simulink model "mrefrobotarm_previous_y_previous_u_previous_ref_cex_2"  (R2018b)
settings: Solver=FixedStepAuto  StartTime=0.0  StopTime=20  RelTol=1e-3  AbsTol=1e-6
undefined symbols (not defined in the file or in its folder): cc, options
libraries: neural x462, simulink x2
(part 16 of 18)

== system mrefrobotarm_previous_y_previous_u_previous_ref_cex_2/no_cex1/Layer 3/Delays 1 ==
  "p{3}" : Inport  PortDimensions=30
      mask Display: e = 0.06;c1 = [120 230 180]/255;c2 = ([120 230 180]+0)/(256+128);c3 = ([120 230 180]+128)/(256+128);patch([0 1 1 0],[0 0 1 1],c1);patch([0 1 1 1-e 1-e 0+e],[0 0 1 1-e 0+e 0+e],c2);patch([0 0 1 1-e 0+e 0+e],[0 1 1 1-e 1-e 0+e],c3);plot([0 1 1 0 0],[0 0 1 1 0]);
  mux : Mux  Inputs=1
      mask Display: e = 0.06;c1 = [120 150 230]/255;c2 = ([120 150 230]+0)/383;c3 = ([120 150 230]+128)/383;patch([0 1 1 0],[0 0 1 1],c1);patch([0 1 1 1-e 1-e 0+e],[0 0 1 1-e 0+e 0+e],c2);patch([0 0 1 1-e 0+e 0+e],[0 1 1 1-e 1-e 0+e],c3);plot([0 1 1 0 0],[0 0 1 1 0]);disp('Mux')
  "pd{3,2}" : Outport
      mask Display: e = 0.06;c1 = [120 230 180]/255;c2 = ([120 230 180]+0)/(256+128);c3 = ([120 230 180]+128)/(256+128);patch([0 1 1 0],[0 0 1 1],c1);patch([0 1 1 1-e 1-e 0+e],[0 0 1 1-e 0+e 0+e],c2);patch([0 0 1 1-e 0+e 0+e],[0 1 1 1-e 1-e 0+e],c3);plot([0 1 1 0 0],[0 0 1 1 0]);
  wires:
  "p{3}"/1 -> mux/1
  mux/1 -> "pd{3,2}"/1

== system mrefrobotarm_previous_y_previous_u_previous_ref_cex_2/no_cex1/Layer 3/LW{3,2} ==
  "ad{3,2}" : Inport  PortDimensions=30
      mask Display: e = 0.06;c1 = [120 230 180]/255;c2 = ([120 230 180]+0)/(256+128);c3 = ([120 230 180]+128)/(256+128);patch([0 1 1 0],[0 0 1 1],c1);patch([0 1 1 1-e 1-e 0+e],[0 0 1 1-e 0+e 0+e],c2);patch([0 0 1 1-e 0+e 0+e],[0 1 1 1-e 1-e 0+e],c3);plot([0 1 1 0 0],[0 0 1 1 0]);
  "IW{3,2}(1,:)'" : Constant  Value=[-0.179633159964680266806880126750911585986614227294921875;-0.01072873765062364037614628387018456123769283294677734375;-0.0291453057248748058360998669513719505630433559417724609375;0.05859045612955075810202032471352140419185161590576171875;-0.237638764700321913903025006220559589564800262451171875;-0.209838527725091539277713081901310943067073822021484375;-0.27791655307496510030063063823035918176174163818359375;-0.07008976059233355815347721318175899796187877655029296875;-0.11554327471293225626514100667918683029711246490478515625;0.27212249906517038677833397741778753697872161865234375;-0.1734031338030869451305449047140427865087985992431640625;0.0536763624525791460673218580268439836800098419189453125;-0.037173437880853761605681739865758572705090045928955078125;0.1358518131119930971717479906146763823926448822021484375;-0.11157815841815578450368917629020870663225650787353515625;-0.023913464068717076027592582931902143172919750213623046875;-0.4313994517536372530486232790281064808368682861328125;0.1636875861604869808463291747102630324661731719970703125;0.037232113811342650022684352961732656694948673248291015625;-0.52644415726454052428806562602403573691844940185546875;0.039897217969779720514456045066253864206373691558837890625;-0.1369287872106144388073545314910006709396839141845703125;0.44593864887069745162051503939437679946422576904296875;0.410742338437982856813590615274733863770961761474609375;-0.145121658875231818175421949490555562078952789306640625;0.06655502995710448066457587401600903831422328948974609375;-0.418109406113754300537976860141498036682605743408203125;0.11096998879556761730125202802810235880315303802490234375;0.333827163986122277261614499366260133683681488037109375;0.186101897373585012385177606120123527944087982177734375]
      mask Display: e = 0.06;c1 = [120 150 230]/255;c2 = ([120 150 230]+0)/383;c3 = ([120 150 230]+128)/383;patch([0 1 1 0],[0 0 1 1],c1);patch([0 1 1 1-e 1-e 0+e],[0 0 1 1-e 0+e 0+e],c2);patch([0 0 1 1-e 0+e 0+e],[0 1 1 1-e 1-e 0+e],c3);plot([0 1 1 0 0],[0 0 1 1 0]);disp('weights');
  Mux : Mux  Inputs=1
      mask Display: e = 0.06;c1 = [120 150 230]/255;c2 = ([120 150 230]+0)/383;c3 = ([120 150 230]+128)/383;patch([0 1 1 0],[0 0 1 1],c1);patch([0 1 1 1-e 1-e 0+e],[0 0 1 1-e 0+e 0+e],c2);patch([0 0 1 1-e 0+e 0+e],[0 1 1 1-e 1-e 0+e],c3);plot([0 1 1 0 0],[0 0 1 1 0]);disp('Mux');
  dotprod1 : neural/Weight Functions/dotprod
  "lz{3,2}" : Outport
      mask Display: e = 0.06;c1 = [120 230 180]/255;c2 = ([120 230 180]+0)/(256+128);c3 = ([120 230 180]+128)/(256+128);patch([0 1 1 0],[0 0 1 1],c1);patch([0 1 1 1-e 1-e 0+e],[0 0 1 1-e 0+e 0+e],c2);patch([0 0 1 1-e 0+e 0+e],[0 1 1 1-e 1-e 0+e],c3);plot([0 1 1 0 0],[0 0 1 1 0]);
  wires:
  "IW{3,2}(1,:)'"/1 -> dotprod1/1
  "ad{3,2}"/1 -> dotprod1/2
  dotprod1/1 -> Mux/1
  Mux/1 -> "lz{3,2}"/1

== system mrefrobotarm_previous_y_previous_u_previous_ref_cex_2/no_cex_old/Layer 1/Delays 1 ==
  "p{1}" : Inport  PortDimensions=10
      mask Display: e = 0.06;c1 = [120 230 180]/255;c2 = ([120 230 180]+0)/(256+128);c3 = ([120 230 180]+128)/(256+128);patch([0 1 1 0],[0 0 1 1],c1);patch([0 1 1 1-e 1-e 0+e],[0 0 1 1-e 0+e 0+e],c2);patch([0 0 1 1-e 0+e 0+e],[0 1 1 1-e 1-e 0+e],c3);plot([0 1 1 0 0],[0 0 1 1 0]);
  mux : Mux  Inputs=1
      mask Display: e = 0.06;c1 = [120 150 230]/255;c2 = ([120 150 230]+0)/383;c3 = ([120 150 230]+128)/383;patch([0 1 1 0],[0 0 1 1],c1);patch([0 1 1 1-e 1-e 0+e],[0 0 1 1-e 0+e 0+e],c2);patch([0 0 1 1-e 0+e 0+e],[0 1 1 1-e 1-e 0+e],c3);plot([0 1 1 0 0],[0 0 1 1 0]);disp('Mux')
  "pd{1,1}" : Outport
      mask Display: e = 0.06;c1 = [120 230 180]/255;c2 = ([120 230 180]+0)/(256+128);c3 = ([120 230 180]+128)/(256+128);patch([0 1 1 0],[0 0 1 1],c1);patch([0 1 1 1-e 1-e 0+e],[0 0 1 1-e 0+e 0+e],c2);patch([0 0 1 1-e 0+e 0+e],[0 1 1 1-e 1-e 0+e],c3);plot([0 1 1 0 0],[0 0 1 1 0]);
  wires:
  "p{1}"/1 -> mux/1
  mux/1 -> "pd{1,1}"/1

== system mrefrobotarm_previous_y_previous_u_previous_ref_cex_2/no_cex_old/Layer 1/IW{1,1} ==
  "pd{1,1}" : Inport  PortDimensions=10
      mask Display: e = 0.06;c1 = [120 230 180]/255;c2 = ([120 230 180]+0)/(256+128);c3 = ([120 230 180]+128)/(256+128);patch([0 1 1 0],[0 0 1 1],c1);patch([0 1 1 1-e 1-e 0+e],[0 0 1 1-e 0+e 0+e],c2);patch([0 0 1 1-e 0+e 0+e],[0 1 1 1-e 1-e 0+e],c3);plot([0 1 1 0 0],[0 0 1 1 0]);
  "IW{1,1}(1,:)'" : Constant  Value=[0.1342886037887657535438989953036070801317691802978515625;-0.145702156505322755197795459025655873119831085205078125;0.05547319335734306189333864267609897069633007049560546875;0.09811034887808976756584655731785460375249385833740234375;-0.115578314062268316941839430000982247292995452880859375;-0.041906530334553958316856636656666523776948451995849609375;0.07401839337125055984234478501093690283596515655517578125;-0.1067335896092770630705359735657111741602420806884765625;0.061760950047272368534923003835501731373369693756103515625;-0.04388287758579813291337501368616358377039432525634765625]
      mask Display: e = 0.06;c1 = [120 150 230]/255;c2 = ([120 150 230]+0)/383;c3 = ([120 150 230]+128)/383;patch([0 1 1 0],[0 0 1 1],c1);patch([0 1 1 1-e 1-e 0+e],[0 0 1 1-e 0+e 0+e],c2);patch([0 0 1 1-e 0+e 0+e],[0 1 1 1-e 1-e 0+e],c3);plot([0 1 1 0 0],[0 0 1 1 0]);disp('Weights');
  "IW{1,1}(10,:)'" : Constant  Value=[-0.00532041249716793014645777049054231611080467700958251953125;0.038558480540163010685805744515164406038820743560791015625;0.038991379228210130969412006152197136543691158294677734375;-0.08418114615032636083302719498533406294882297515869140625;0.213756443707833587719591150744236074388027191162109375;0.1686868532677217313864304060189169831573963165283203125;0.2339894746184230378549528950316016562283039093017578125;0.1786960217132106676363179076361120678484439849853515625;0.171502593476762277280300850179628469049930572509765625;0.0182816548613749761675872917976448661647737026214599609375]
      mask Display: e = 0.06;c1 = [120 150 230]/255;c2 = ([120 150 230]+0)/383;c3 = ([120 150 230]+128)/383;patch([0 1 1 0],[0 0 1 1],c1);patch([0 1 1 1-e 1-e 0+e],[0 0 1 1-e 0+e 0+e],c2);patch([0 0 1 1-e 0+e 0+e],[0 1 1 1-e 1-e 0+e],c3);plot([0 1 1 0 0],[0 0 1 1 0]);disp('Weights');
  "IW{1,1}(11,:)'" : Constant  Value=[0.035705063792069495487435659697439405135810375213623046875;0.1307324517390685281181816890239133499562740325927734375;-0.04209371294231502302896075207172543741762638092041015625;-0.1389322563683020594904604649855173192918300628662109375;0.11087205351285255028326304227448417805135250091552734375;-0.02149692902052637022425329860197962261736392974853515625;-0.031691065556913623757484543830287293531000614166259765625;-0.148095139947966802917989070920157246291637420654296875;0.13326976965195125313101698338869027793407440185546875;-0.039387551991871376511067381898101302795112133026123046875]
      mask Display: e = 0.06;c1 = [120 150 230]/255;c2 = ([120 150 230]+0)/383;c3 = ([120 150 230]+128)/383;patch([0 1 1 0],[0 0 1 1],c1);patch([0 1 1 1-e 1-e 0+e],[0 0 1 1-e 0+e 0+e],c2);patch([0 0 1 1-e 0+e 0+e],[0 1 1 1-e 1-e 0+e],c3);plot([0 1 1 0 0],[0 0 1 1 0]);disp('Weights');
  "IW{1,1}(12,:)'" : Constant  Value=[0.0963310683293380487501877951217466033995151519775390625;-0.1696662291031194869095344301967998035252094268798828125;0.077263620014577816252909769900725223124027252197265625;0.006392641361406257473343206498839208506979048252105712890625;-0.03771605055298239694838713376157102175056934356689453125;-0.0243720968334742958683047930890097632072865962982177734375;0.039947602899256529074278887492255307734012603759765625;0.018849788000436872026366330601376830600202083587646484375;-0.09559877755313206382226098867249675095081329345703125;0.11457489976111269458503016949180164374411106109619140625]
      mask Display: e = 0.06;c1 = [120 150 230]/255;c2 = ([120 150 230]+0)/383;c3 = ([120 150 230]+128)/383;patch([0 1 1 0],[0 0 1 1],c1);patch([0 1 1 1-e 1-e 0+e],[0 0 1 1-e 0+e 0+e],c2);patch([0 0 1 1-e 0+e 0+e],[0 1 1 1-e 1-e 0+e],c3);plot([0 1 1 0 0],[0 0 1 1 0]);disp('Weights');
  "IW{1,1}(13,:)'" : Constant  Value=[-0.170367891135734750296393258395255543291568756103515625;0.1690618062897462359206457449545268900692462921142578125;-0.0679022999928180770456975778870400972664356231689453125;0.0567564025005189154438056675644475035369396209716796875;-0.10659871075086345404425713923046714626252651214599609375;-0.2552475580253259490604023085325025022029876708984375;0.1578920500425812500910893731997930444777011871337890625;0.007230833901438897363955771169230501982383430004119873046875;0.01262097650695703961176707963431908865459263324737548828125;-0.07259975591463964372795913959635072387754917144775390625]
      mask Display: e = 0.06;c1 = [120 150 230]/255;c2 = ([120 150 230]+0)/383;c3 = ([120 150 230]+128)/383;patch([0 1 1 0],[0 0 1 1],c1);patch([0 1 1 1-e 1-e 0+e],[0 0 1 1-e 0+e 0+e],c2);patch([0 0 1 1-e 0+e 0+e],[0 1 1 1-e 1-e 0+e],c3);plot([0 1 1 0 0],[0 0 1 1 0]);disp('Weights');
  "IW{1,1}(14,:)'" : Constant  Value=[0.06474261454726214226607083901399164460599422454833984375;-0.11509349165920192137324562509093084372580051422119140625;-0.11350537964576583316311797489106538705527782440185546875;0.1523399415267104040072609905109857209026813507080078125;-0.14329360609649854918501432621269486844539642333984375;0.14377878539324928652831658837385475635528564453125;-0.0168196406057015586388292405217725900001823902130126953125;-0.01416279737589609157011327766895192326046526432037353515625;-0.0289317569535016104464997255263369879685342311859130859375;0.11819705598629139109423391573727712966501712799072265625]
      mask Display: e = 0.06;c1 = [120 150 230]/255;c2 = ([120 150 230]+0)/383;c3 = ([120 150 230]+128)/383;patch([0 1 1 0],[0 0 1 1],c1);patch([0 1 1 1-e 1-e 0+e],[0 0 1 1-e 0+e 0+e],c2);patch([0 0 1 1-e 0+e 0+e],[0 1 1 1-e 1-e 0+e],c3);plot([0 1 1 0 0],[0 0 1 1 0]);disp('Weights');
  "IW{1,1}(15,:)'" : Constant  Value=[0.02213412452375995709275002809590660035610198974609375;0.0194307297856310366712673243227982311509549617767333984375;0.05936634958668797479308665288044721819460391998291015625;-0.227109536896744013123594641001545824110507965087890625;-0.059328902646757476768701877745115780271589756011962890625;0.0239874165518910442695954543523839674890041351318359375;-0.0124729668598871253071269649126406875438988208770751953125;-0.1523221403384991956553307090871385298669338226318359375;-0.00885500118978834772909269901219886378385126590728759765625;0.03748756183767758265457104016604716889560222625732421875]
      mask Display: e = 0.06;c1 = [120 150 230]/255;c2 = ([120 150 230]+0)/383;c3 = ([120 150 230]+128)/383;patch([0 1 1 0],[0 0 1 1],c1);patch([0 1 1 1-e 1-e 0+e],[0 0 1 1-e 0+e 0+e],c2);patch([0 0 1 1-e 0+e 0+e],[0 1 1 1-e 1-e 0+e],c3);plot([0 1 1 0 0],[0 0 1 1 0]);disp('Weights');
  "IW{1,1}(16,:)'" : Constant  Value=[-0.069668964603038452398919844199554063379764556884765625;0.309683875764699856336648053911630995571613311767578125;-0.2120492827081727205129624280743882991373538970947265625;0.005686553722663730513209312533717820770107209682464599609375;0.2860354896080867792562685281154699623584747314453125;-0.449590820638774035788998162388452328741550445556640625;0.2170978996645353820138524270078050903975963592529296875;-0.00962913152344563490203643851828019251115620136260986328125;-0.136743780075903209603183086073840968310832977294921875;-0.341127538317710421456041558485594578087329864501953125]
      mask Display: e = 0.06;c1 = [120 150 230]/255;c2 = ([120 150 230]+0)/383;c3 = ([120 150 230]+128)/383;patch([0 1 1 0],[0 0 1 1],c1);patch([0 1 1 1-e 1-e 0+e],[0 0 1 1-e 0+e 0+e],c2);patch([0 0 1 1-e 0+e 0+e],[0 1 1 1-e 1-e 0+e],c3);plot([0 1 1 0 0],[0 0 1 1 0]);disp('Weights');
  "IW{1,1}(17,:)'" : Constant  Value=[-0.09825337350828979021688525108402245678007602691650390625;-0.1890337654701977621041208976748748682439327239990234375;0.046160009121197165260497285999008454382419586181640625;0.09385000156687682559830676609635702334344387054443359375;-0.11448783645044686985148274516177480109035968780517578125;-0.1102885778507775860202144713184679858386516571044921875;-0.27756559899467114771454134825034998357295989990234375;-0.241301771620663296769038197453483007848262786865234375;0.0270645110259145928177648698920165770687162876129150390625;0.045580012746472602092051573663411545567214488983154296875]
      mask Display: e = 0.06;c1 = [120 150 230]/255;c2 = ([120 150 230]+0)/383;c3 = ([120 150 230]+128)/383;patch([0 1 1 0],[0 0 1 1],c1);patch([0 1 1 1-e 1-e 0+e],[0 0 1 1-e 0+e 0+e],c2);patch([0 0 1 1-e 0+e 0+e],[0 1 1 1-e 1-e 0+e],c3);plot([0 1 1 0 0],[0 0 1 1 0]);disp('Weights');
  "IW{1,1}(18,:)'" : Constant  Value=[-0.1593685780621468539575147360665141604840755462646484375;-0.061281035001929155814348604280894505791366100311279296875;0.056944711965067063008660852574394084513187408447265625;0.182778738498478088292387155888718552887439727783203125;0.1801621464179990750320570214171311818063259124755859375;0.1508937474301184356040295142520335502922534942626953125;0.1853260785695341750223263943553320132195949554443359375;0.09317688804506769895130702252572518773376941680908203125;0.11313555617204411329890234583217534236609935760498046875;-0.194719394756256936052096762068686075508594512939453125]
      mask Display: e = 0.06;c1 = [120 150 230]/255;c2 = ([120 150 230]+0)/383;c3 = ([120 150 230]+128)/383;patch([0 1 1 0],[0 0 1 1],c1);patch([0 1 1 1-e 1-e 0+e],[0 0 1 1-e 0+e 0+e],c2);patch([0 0 1 1-e 0+e 0+e],[0 1 1 1-e 1-e 0+e],c3);plot([0 1 1 0 0],[0 0 1 1 0]);disp('Weights');
  "IW{1,1}(19,:)'" : Constant  Value=[0.057079349368471636594346563242652337066829204559326171875;-0.1296401607201551897663449608444352634251117706298828125;-0.031371944496909977273535474751042784191668033599853515625;0.09029385696961565732632237768484628759324550628662109375;-0.001802648021193855275290385264952419674955308437347412109375;-0.07192536237898801421142280787535128183662891387939453125;0.03904728530171790168434853285361896269023418426513671875;-0.1544853968620005790768345832475461065769195556640625;0.09921966980443340522466399988843477331101894378662109375;-0.066942021458685607715466403533355332911014556884765625]
      mask Display: e = 0.06;c1 = [120 150 230]/255;c2 = ([120 150 230]+0)/383;c3 = ([120 150 230]+128)/383;patch([0 1 1 0],[0 0 1 1],c1);patch([0 1 1 1-e 1-e 0+e],[0 0 1 1-e 0+e 0+e],c2);patch([0 0 1 1-e 0+e 0+e],[0 1 1 1-e 1-e 0+e],c3);plot([0 1 1 0 0],[0 0 1 1 0]);disp('Weights');
  "IW{1,1}(2,:)'" : Constant  Value=[0.07242176646470781242737047023183549754321575164794921875;0.1049414314609020404400752113360795192420482635498046875;0.1712039638627951554372685905036632902920246124267578125;0.18599232490624373337340102807502262294292449951171875;0.1124116274754447253325650990518624894320964813232421875;0.00851940589409703151468900017562191351316869258880615234375;0.1285194531608742363193442770352703519165515899658203125;0.0284037291034748388962594134454775485210120677947998046875;-0.006873467381939313801397783976199207245372235774993896484375;-0.0281291352428563630472257983683448401279747486114501953125]
      mask Display: e = 0.06;c1 = [120 150 230]/255;c2 = ([120 150 230]+0)/383;c3 = ([120 150 230]+128)/383;patch([0 1 1 0],[0 0 1 1],c1);patch([0 1 1 1-e 1-e 0+e],[0 0 1 1-e 0+e 0+e],c2);patch([0 0 1 1-e 0+e 0+e],[0 1 1 1-e 1-e 0+e],c3);plot([0 1 1 0 0],[0 0 1 1 0]);disp('Weights');
  "IW{1,1}(20,:)'" : Constant  Value=[0.00435123337447600178062856457472662441432476043701171875;0.10977328237297302726549474982675747014582157135009765625;-0.03832069334747680022790206066929385997354984283447265625;0.08732543865773025049126232488561072386801242828369140625;-0.1286192632937832869277627878545899875462055206298828125;-0.1096816005171722119282406993079348467290401458740234375;-0.181385739328361328404071173281408846378326416015625;-0.1383045483001802133937729877288802526891231536865234375;-0.0678912866207693477260676218065782450139522552490234375;-0.057390197085697751411270672861064667813479900360107421875]
      mask Display: e = 0.06;c1 = [120 150 230]/255;c2 = ([120 150 230]+0)/383;c3 = ([120 150 230]+128)/383;patch([0 1 1 0],[0 0 1 1],c1);patch([0 1 1 1-e 1-e 0+e],[0 0 1 1-e 0+e 0+e],c2);patch([0 0 1 1-e 0+e 0+e],[0 1 1 1-e 1-e 0+e],c3);plot([0 1 1 0 0],[0 0 1 1 0]);disp('Weights');
  "IW{1,1}(21,:)'" : Constant  Value=[-0.01410806149226366025539736170912874513305723667144775390625;0.1328917351620661768674125369216199032962322235107421875;-0.06271456621733086100878296065275208093225955963134765625;0.054189716251180797268460764826158992946147918701171875;0.0590676698905578945186789496801793575286865234375;0.06621089359857522393948414674014202319085597991943359375;0.1058392442421232371163597463237238116562366485595703125;-0.00851306153757265364478978852957880008034408092498779296875;0.09854766233504171080159750317761790938675403594970703125;0.09899106591023611179114283231683657504618167877197265625]
      mask Display: e = 0.06;c1 = [120 150 230]/255;c2 = ([120 150 230]+0)/383;c3 = ([120 150 230]+128)/383;patch([0 1 1 0],[0 0 1 1],c1);patch([0 1 1 1-e 1-e 0+e],[0 0 1 1-e 0+e 0+e],c2);patch([0 0 1 1-e 0+e 0+e],[0 1 1 1-e 1-e 0+e],c3);plot([0 1 1 0 0],[0 0 1 1 0]);disp('Weights');
  "IW{1,1}(22,:)'" : Constant  Value=[-0.054294408303833412154926207904281909577548503875732421875;0.14154556325499079161289728290284983813762664794921875;-0.10956781139197734054047117524532950483262538909912109375;-0.07051200545425105603580817614783882163465023040771484375;0.1372632548900360738297621310266549699008464813232421875;-0.1216287955921996621899694446256035007536411285400390625;0.08081288046265037994242419472357141785323619842529296875;0.09711299986610590073699000868145958520472049713134765625;0.027426365671638384957642387007581419311463832855224609375;0.07208448672155996772570318853468052111566066741943359375]
      mask Display: e = 0.06;c1 = [120 150 230]/255;c2 = ([120 150 230]+0)/383;c3 = ([120 150 230]+128)/383;patch([0 1 1 0],[0 0 1 1],c1);patch([0 1 1 1-e 1-e 0+e],[0 0 1 1-e 0+e 0+e],c2);patch([0 0 1 1-e 0+e 0+e],[0 1 1 1-e 1-e 0+e],c3);plot([0 1 1 0 0],[0 0 1 1 0]);disp('Weights');
  "IW{1,1}(23,:)'" : Constant  Value=[0.07330337518800934815121905785417766310274600982666015625;-0.00394633378621255838381021163741024793125689029693603515625;-0.03155610514682870293423633256679750047624111175537109375;0.040880253327475468694274240988306701183319091796875;0.037118320947610132509719704785311478190124034881591796875;0.07764536240814161327516984556496026925742626190185546875;0.15422657826953434234695805571391247212886810302734375;-0.07559617315376167268059504067423404194414615631103515625;0.08586977940837432765608383533617598004639148712158203125;-0.08664417960724579703679637532331980764865875244140625]
      mask Display: e = 0.06;c1 = [120 150 230]/255;c2 = ([120 150 230]+0)/383;c3 = ([120 150 230]+128)/383;patch([0 1 1 0],[0 0 1 1],c1);patch([0 1 1 1-e 1-e 0+e],[0 0 1 1-e 0+e 0+e],c2);patch([0 0 1 1-e 0+e 0+e],[0 1 1 1-e 1-e 0+e],c3);plot([0 1 1 0 0],[0 0 1 1 0]);disp('Weights');
  "IW{1,1}(24,:)'" : Constant  Value=[0.2184359879879601840091396525167510844767093658447265625;-0.059007570758309278724507151991929276846349239349365234375;0.09354525549086699365286534657570882700383663177490234375;-0.0772961168694774602982988653820939362049102783203125;0.06665430207182894417616836335582775063812732696533203125;0.09492169145886118764021688321008696220815181732177734375;-0.0653790025735966617848049509120755828917026519775390625;0.052988817636760755791502930378555902279913425445556640625;-0.1284011701573265773479448625948862172663211822509765625;0.018580750903621316705294219673305633477866649627685546875]
      mask Display: e = 0.06;c1 = [120 150 230]/255;c2 = ([120 150 230]+0)/383;c3 = ([120 150 230]+128)/383;patch([0 1 1 0],[0 0 1 1],c1);patch([0 1 1 1-e 1-e 0+e],[0 0 1 1-e 0+e 0+e],c2);patch([0 0 1 1-e 0+e 0+e],[0 1 1 1-e 1-e 0+e],c3);plot([0 1 1 0 0],[0 0 1 1 0]);disp('Weights');
  "IW{1,1}(25,:)'" : Constant  Value=[0.0675656852302155552791873560636304318904876708984375;-0.1327295511201762590047792400582693517208099365234375;-0.08002107763594239198123858614053460769355297088623046875;0.10203247506578783099229212893988005816936492919921875;-0.1028463726444479586774605195387266576290130615234375;-0.060949980848724653881287594003879348747432231903076171875;0.07472279567773841557620784215032472275197505950927734375;0.06751254914899999792776696949658798985183238983154296875;-0.06159377004665202159916503887870931066572666168212890625;-0.0554695333338589835481258205618360079824924468994140625]
      mask Display: e = 0.06;c1 = [120 150 230]/255;c2 = ([120 150 230]+0)/383;c3 = ([120 150 230]+128)/383;patch([0 1 1 0],[0 0 1 1],c1);patch([0 1 1 1-e 1-e 0+e],[0 0 1 1-e 0+e 0+e],c2);patch([0 0 1 1-e 0+e 0+e],[0 1 1 1-e 1-e 0+e],c3);plot([0 1 1 0 0],[0 0 1 1 0]);disp('Weights');
  "IW{1,1}(26,:)'" : Constant  Value=[0.1703437559283320357206292783303069882094860076904296875;0.092992374667536681354107486185966990888118743896484375;0.16302848740754516398965279222466051578521728515625;0.110211383534811691031762848069774918258190155029296875;0.044276127259902479937903052586989360861480236053466796875;-0.05558661417890757572290993948627146892249584197998046875;0.0284198468833597762961407084958409541286528110504150390625;-0.1440396494869803090121962441116920672357082366943359375;-0.09076978451211592524572324691689573228359222412109375;0.056235840684018024993040540948641137219965457916259765625]
      mask Display: e = 0.06;c1 = [120 150 230]/255;c2 = ([120 150 230]+0)/383;c3 = ([120 150 230]+128)/383;patch([0 1 1 0],[0 0 1 1],c1);patch([0 1 1 1-e 1-e 0+e],[0 0 1 1-e 0+e 0+e],c2);patch([0 0 1 1-e 0+e 0+e],[0 1 1 1-e 1-e 0+e],c3);plot([0 1 1 0 0],[0 0 1 1 0]);disp('Weights');
  "IW{1,1}(27,:)'" : Constant  Value=[-0.1671222824114687310892435334608308039605617523193359375;0.0734579551130998265051630369271151721477508544921875;-0.121440951396859009303597076723235659301280975341796875;-0.052447262216427405212559875735678360797464847564697265625;0.13464667957406983855861426491173915565013885498046875;-0.017565097138921660635535459960010484792292118072509765625;-0.0579655644317933482767557507031597197055816650390625;0.01209289287151457496782835931981026078574359416961669921875;0.002460803272943997387078862715270588523708283901214599609375;0.0634301892291257163325468582115718163549900054931640625]
      mask Display: e = 0.06;c1 = [120 150 230]/255;c2 = ([120 150 230]+0)/383;c3 = ([120 150 230]+128)/383;patch([0 1 1 0],[0 0 1 1],c1);patch([0 1 1 1-e 1-e 0+e],[0 0 1 1-e 0+e 0+e],c2);patch([0 0 1 1-e 0+e 0+e],[0 1 1 1-e 1-e 0+e],c3);plot([0 1 1 0 0],[0 0 1 1 0]);disp('Weights');
  "IW{1,1}(28,:)'" : Constant  Value=[0.151517403982598997114195071844733320176601409912109375;0.1153440450307792464190725922890123911201953887939453125;0.165914688874000015861298606978380121290683746337890625;0.1769233504277152035921716333177755586802959442138671875;0.11562785316669550728096993452709284611046314239501953125;0.0713206898896436014556599047864438034594058990478515625;0.0010539916827221186383656270635356122511439025402069091796875;0.1402354116991490762256233892912860028445720672607421875;0.08767505292549455930828372629548539407551288604736328125;-0.1187254458494778897037491560695343650877475738525390625]
      mask Display: e = 0.06;c1 = [120 150 230]/255;c2 = ([120 150 230]+0)/383;c3 = ([120 150 230]+128)/383;patch([0 1 1 0],[0 0 1 1],c1);patch([0 1 1 1-e 1-e 0+e],[0 0 1 1-e 0+e 0+e],c2);patch([0 0 1 1-e 0+e 0+e],[0 1 1 1-e 1-e 0+e],c3);plot([0 1 1 0 0],[0 0 1 1 0]);disp('Weights');
  "IW{1,1}(29,:)'" : Constant  Value=[-0.1709566132488007095258097933765384368598461151123046875;0.139729105844223877586074422652018256485462188720703125;-0.01063970597820372565589508440098143182694911956787109375;-0.02826720609368636727420920351505628786981105804443359375;-0.057269493589525814758456334629954653792083263397216796875;-0.1206518476189940292098157215150422416627407073974609375;0.09153989056150686753898781944371876306831836700439453125;-0.08799750888187586606026258095880621112883090972900390625;0.0017290181057740138144407371356692237895913422107696533203125;-0.0013240483020594668271685545590798938064835965633392333984375]
      mask Display: e = 0.06;c1 = [120 150 230]/255;c2 = ([120 150 230]+0)/383;c3 = ([120 150 230]+128)/383;patch([0 1 1 0],[0 0 1 1],c1);patch([0 1 1 1-e 1-e 0+e],[0 0 1 1-e 0+e 0+e],c2);patch([0 0 1 1-e 0+e 0+e],[0 1 1 1-e 1-e 0+e],c3);plot([0 1 1 0 0],[0 0 1 1 0]);disp('Weights');
  "IW{1,1}(3,:)'" : Constant  Value=[-0.214456259135830940021349988455767743289470672607421875;-0.036116213738735282456904229775318526662886142730712890625;0.0217965632429515006329712178967383806593716144561767578125;-0.109082564991107966445582633241428993642330169677734375;0.06912590938770428461435102462928625755012035369873046875;0.0107361858131412545025451521496506757102906703948974609375;-0.014725477066765170486295488672112696804106235504150390625;-0.05476680503146884315679443488988908939063549041748046875;-0.025498292591681494256850015744930715300142765045166015625;0.0850838897551909056904406725152512080967426300048828125]
      mask Display: e = 0.06;c1 = [120 150 230]/255;c2 = ([120 150 230]+0)/383;c3 = ([120 150 230]+128)/383;patch([0 1 1 0],[0 0 1 1],c1);patch([0 1 1 1-e 1-e 0+e],[0 0 1 1-e 0+e 0+e],c2);patch([0 0 1 1-e 0+e 0+e],[0 1 1 1-e 1-e 0+e],c3);plot([0 1 1 0 0],[0 0 1 1 0]);disp('Weights');
  "IW{1,1}(30,:)'" : Constant  Value=[-0.140459566567950833171352087447303347289562225341796875;0.12388115316699492562957374275356414727866649627685546875;-0.0124581242070213767114683633963068132288753986358642578125;-0.04607145461452370749366735935836913995444774627685546875;-0.04540432285834473946639633368249633349478244781494140625;-0.180571072300906576568735317778191529214382171630859375;0.10631755317234174718077355237255687825381755828857421875;0.059826757456727254480544075931902625598013401031494140625;-0.05559491306193041493255435625542304478585720062255859375;-0.1131211289932436414584771000590990297496318817138671875]
      mask Display: e = 0.06;c1 = [120 150 230]/255;c2 = ([120 150 230]+0)/383;c3 = ([120 150 230]+128)/383;patch([0 1 1 0],[0 0 1 1],c1);patch([0 1 1 1-e 1-e 0+e],[0 0 1 1-e 0+e 0+e],c2);patch([0 0 1 1-e 0+e 0+e],[0 1 1 1-e 1-e 0+e],c3);plot([0 1 1 0 0],[0 0 1 1 0]);disp('Weights');
  "IW{1,1}(4,:)'" : Constant  Value=[-0.165879169192116593389840772942989133298397064208984375;-0.0893536879525311800165354725322686135768890380859375;-0.06315669959565496649478433255353593267500400543212890625;0.01928780999598601886280135886408970691263675689697265625;0.03745120053701984919047873745512333698570728302001953125;0.1707491879389413103051964526457595638930797576904296875;0.0877189124274228848587853235585498623549938201904296875;0.1761829839069997405420764380323817022144794464111328125;-0.01010316150119708843158061739586628391407430171966552734375;0.000971025483142991794639764524532665745937265455722808837890625]
      mask Display: e = 0.06;c1 = [120 150 230]/255;c2 = ([120 150 230]+0)/383;c3 = ([120 150 230]+128)/383;patch([0 1 1 0],[0 0 1 1],c1);patch([0 1 1 1-e 1-e 0+e],[0 0 1 1-e 0+e 0+e],c2);patch([0 0 1 1-e 0+e 0+e],[0 1 1 1-e 1-e 0+e],c3);plot([0 1 1 0 0],[0 0 1 1 0]);disp('Weights');
  "IW{1,1}(5,:)'" : Constant  Value=[-0.1164692117417917838206875558171304874122142791748046875;-0.1549484328329745197461164707419811747968196868896484375;0.081154072111970954050974569327081553637981414794921875;0.163378442341789220648706759675405919551849365234375;0.115034213959365139157142721160198561847209930419921875;0.054312077850814412249835783086382434703409671783447265625;-0.103870604431010427060044776226277463138103485107421875;-0.0496174334665817340361826381922583095729351043701171875;-0.1748364037026159667487235083171981386840343475341796875;-0.0571351632795144281917743001031340099871158599853515625]
      mask Display: e = 0.06;c1 = [120 150 230]/255;c2 = ([120 150 230]+0)/383;c3 = ([120 150 230]+128)/383;patch([0 1 1 0],[0 0 1 1],c1);patch([0 1 1 1-e 1-e 0+e],[0 0 1 1-e 0+e 0+e],c2);patch([0 0 1 1-e 0+e 0+e],[0 1 1 1-e 1-e 0+e],c3);plot([0 1 1 0 0],[0 0 1 1 0]);disp('Weights');
  "IW{1,1}(6,:)'" : Constant  Value=[0.1382699523442445233012421113016898743808269500732421875;0.047666816400552487753561337058272329159080982208251953125;-0.06827729944410441953461798902935697697103023529052734375;0.06385874299566761391755420618210337124764919281005859375;0.1300406183707694951490196899612783454358577728271484375;0.10202829458648639271434177544506383128464221954345703125;-0.0537156829829590065639166596156428568065166473388671875;0.03550303192659372275574725108526763506233692169189453125;-0.09636868904922822609560029150088666938245296478271484375;0.09993030347911190103271650286842486821115016937255859375]
      mask Display: e = 0.06;c1 = [120 150 230]/255;c2 = ([120 150 230]+0)/383;c3 = ([120 150 230]+128)/383;patch([0 1 1 0],[0 0 1 1],c1);patch([0 1 1 1-e 1-e 0+e],[0 0 1 1-e 0+e 0+e],c2);patch([0 0 1 1-e 0+e 0+e],[0 1 1 1-e 1-e 0+e],c3);plot([0 1 1 0 0],[0 0 1 1 0]);disp('Weights');
  "IW{1,1}(7,:)'" : Constant  Value=[0.038868996926507838607367517624879837967455387115478515625;-0.1410080132101939887068198231645510531961917877197265625;0.0868322409872927802876318992275628261268138885498046875;-0.0782188967970567083920485629278118722140789031982421875;-0.07782057967372076057177565644451533444225788116455078125;0.056062646289928748377651146483913180418312549591064453125;-0.064890175549565665136242387234233319759368896484375;-0.0029371144154630309495990214685434693819843232631683349609375;-0.045874046978748077296739182884266483597457408905029296875;0.15071513215093446103054475315730087459087371826171875]
      mask Display: e = 0.06;c1 = [120 150 230]/255;c2 = ([120 150 230]+0)/383;c3 = ([120 150 230]+128)/383;patch([0 1 1 0],[0 0 1 1],c1);patch([0 1 1 1-e 1-e 0+e],[0 0 1 1-e 0+e 0+e],c2);patch([0 0 1 1-e 0+e 0+e],[0 1 1 1-e 1-e 0+e],c3);plot([0 1 1 0 0],[0 0 1 1 0]);disp('Weights');
  "IW{1,1}(8,:)'" : Constant  Value=[-0.035236812752056569097991456374074914492666721343994140625;-0.06327595241940543735470470210202620364725589752197265625;-0.124917664151006524431153366094804368913173675537109375;-0.1174108520552865631003669477649964392185211181640625;-0.1413183540559711237616369317038333974778652191162109375;-0.0430230556547836762160130774645949713885784149169921875;-0.03948134555601638673305586735295946709811687469482421875;0.1205758971064148088458978236303664743900299072265625;0.0294993587841617839473418172246965696103870868682861328125;0.0159887100690661275448345435279406956396996974945068359375]
      mask Display: e = 0.06;c1 = [120 150 230]/255;c2 = ([120 150 230]+0)/383;c3 = ([120 150 230]+128)/383;patch([0 1 1 0],[0 0 1 1],c1);patch([0 1 1 1-e 1-e 0+e],[0 0 1 1-e 0+e 0+e],c2);patch([0 0 1 1-e 0+e 0+e],[0 1 1 1-e 1-e 0+e],c3);plot([0 1 1 0 0],[0 0 1 1 0]);disp('Weights');
  "IW{1,1}(9,:)'" : Constant  Value=[-0.08887942344159506513623369983179145492613315582275390625;0.190470197165957255691637328709475696086883544921875;-0.05516951157718129328255685095427907072007656097412109375;0.07253289572917076544200654097949154675006866455078125;0.07587440809784050388397957931374548934400081634521484375;-0.08369413535223317601730030901308055035769939422607421875;-0.01298159792138756270241106705043421243317425251007080078125;-0.08030203834624881353843051101648597978055477142333984375;0.0214418889397328983614787745182184153236448764801025390625;-0.146549967054692420465045188393560238182544708251953125]
      mask Display: e = 0.06;c1 = [120 150 230]/255;c2 = ([120 150 230]+0)/383;c3 = ([120 150 230]+128)/383;patch([0 1 1 0],[0 0 1 1],c1);patch([0 1 1 1-e 1-e 0+e],[0 0 1 1-e 0+e 0+e],c2);patch([0 0 1 1-e 0+e 0+e],[0 1 1 1-e 1-e 0+e],c3);plot([0 1 1 0 0],[0 0 1 1 0]);disp('Weights');
  Mux : Mux  Inputs=30
      mask Display: e = 0.06;c1 = [120 150 230]/255;c2 = ([120 150 230]+0)/383;c3 = ([120 150 230]+128)/383;patch([0 1 1 0],[0 0 1 1],c1);patch([0 1 1 1-e 1-e 0+e],[0 0 1 1-e 0+e 0+e],c2);patch([0 0 1 1-e 0+e 0+e],[0 1 1 1-e 1-e 0+e],c3);plot([0 1 1 0 0],[0 0 1 1 0]);disp('Mux');
  dotprod{1..30} (30 alike) : neural/Weight Functions/dotprod
  "iz{1,1}" : Outport
      mask Display: e = 0.06;c1 = [120 230 180]/255;c2 = ([120 230 180]+0)/(256+128);c3 = ([120 230 180]+128)/(256+128);patch([0 1 1 0],[0 0 1 1],c1);patch([0 1 1 1-e 1-e 0+e],[0 0 1 1-e 0+e 0+e],c2);patch([0 0 1 1-e 0+e 0+e],[0 1 1 1-e 1-e 0+e],c3);plot([0 1 1 0 0],[0 0 1 1 0]);
  wires:
  "IW{1,1}(1,:)'"/1 -> dotprod1/1
  "pd{1,1}"/1 -> dotprod1/2, dotprod2/2, dotprod3/2, dotprod4/2, dotprod5/2, dotprod6/2, dotprod7/2, dotprod8/2, dotprod9/2, dotprod10/2, dotprod11/2, dotprod12/2, dotprod13/2, dotprod14/2, dotprod15/2, dotprod16/2, dotprod17/2, dotprod18/2, dotprod19/2, dotprod20/2, dotprod21/2, dotprod22/2, dotprod23/2, dotprod24/2, dotprod25/2, dotprod26/2, dotprod27/2, dotprod28/2, dotprod29/2, dotprod30/2
  dotprod1/1 -> Mux/1
  "IW{1,1}(2,:)'"/1 -> dotprod2/1
  dotprod2/1 -> Mux/2
  "IW{1,1}(3,:)'"/1 -> dotprod3/1
  dotprod3/1 -> Mux/3
  "IW{1,1}(4,:)'"/1 -> dotprod4/1
  dotprod4/1 -> Mux/4
  "IW{1,1}(5,:)'"/1 -> dotprod5/1
  dotprod5/1 -> Mux/5
  "IW{1,1}(6,:)'"/1 -> dotprod6/1
  dotprod6/1 -> Mux/6
  "IW{1,1}(7,:)'"/1 -> dotprod7/1
  dotprod7/1 -> Mux/7
  "IW{1,1}(8,:)'"/1 -> dotprod8/1
  dotprod8/1 -> Mux/8
  "IW{1,1}(9,:)'"/1 -> dotprod9/1
  dotprod9/1 -> Mux/9
  "IW{1,1}(10,:)'"/1 -> dotprod10/1
  dotprod10/1 -> Mux/10
  "IW{1,1}(11,:)'"/1 -> dotprod11/1
  dotprod11/1 -> Mux/11
  "IW{1,1}(12,:)'"/1 -> dotprod12/1
  dotprod12/1 -> Mux/12
  "IW{1,1}(13,:)'"/1 -> dotprod13/1
  dotprod13/1 -> Mux/13
  "IW{1,1}(14,:)'"/1 -> dotprod14/1
  dotprod14/1 -> Mux/14
  "IW{1,1}(15,:)'"/1 -> dotprod15/1
  dotprod15/1 -> Mux/15
  "IW{1,1}(16,:)'"/1 -> dotprod16/1
  dotprod16/1 -> Mux/16
  "IW{1,1}(17,:)'"/1 -> dotprod17/1
  dotprod17/1 -> Mux/17
  "IW{1,1}(18,:)'"/1 -> dotprod18/1
  dotprod18/1 -> Mux/18
  "IW{1,1}(19,:)'"/1 -> dotprod19/1
  dotprod19/1 -> Mux/19
  "IW{1,1}(20,:)'"/1 -> dotprod20/1
  dotprod20/1 -> Mux/20
  "IW{1,1}(21,:)'"/1 -> dotprod21/1
  dotprod21/1 -> Mux/21
  "IW{1,1}(22,:)'"/1 -> dotprod22/1
  dotprod22/1 -> Mux/22
  "IW{1,1}(23,:)'"/1 -> dotprod23/1
  dotprod23/1 -> Mux/23
  "IW{1,1}(24,:)'"/1 -> dotprod24/1
  dotprod24/1 -> Mux/24
  "IW{1,1}(25,:)'"/1 -> dotprod25/1
  dotprod25/1 -> Mux/25
  "IW{1,1}(26,:)'"/1 -> dotprod26/1
  dotprod26/1 -> Mux/26
  "IW{1,1}(27,:)'"/1 -> dotprod27/1
  dotprod27/1 -> Mux/27
  "IW{1,1}(28,:)'"/1 -> dotprod28/1
  dotprod28/1 -> Mux/28
  "IW{1,1}(29,:)'"/1 -> dotprod29/1
  dotprod29/1 -> Mux/29
  "IW{1,1}(30,:)'"/1 -> dotprod30/1
  dotprod30/1 -> Mux/30
  Mux/1 -> "iz{1,1}"/1

== system mrefrobotarm_previous_y_previous_u_previous_ref_cex_2/no_cex_old/Layer 2/Delays 1 ==
  "p{2}" : Inport  PortDimensions=30
      mask Display: e = 0.06;c1 = [120 230 180]/255;c2 = ([120 230 180]+0)/(256+128);c3 = ([120 230 180]+128)/(256+128);patch([0 1 1 0],[0 0 1 1],c1);patch([0 1 1 1-e 1-e 0+e],[0 0 1 1-e 0+e 0+e],c2);patch([0 0 1 1-e 0+e 0+e],[0 1 1 1-e 1-e 0+e],c3);plot([0 1 1 0 0],[0 0 1 1 0]);
  mux : Mux  Inputs=1
      mask Display: e = 0.06;c1 = [120 150 230]/255;c2 = ([120 150 230]+0)/383;c3 = ([120 150 230]+128)/383;patch([0 1 1 0],[0 0 1 1],c1);patch([0 1 1 1-e 1-e 0+e],[0 0 1 1-e 0+e 0+e],c2);patch([0 0 1 1-e 0+e 0+e],[0 1 1 1-e 1-e 0+e],c3);plot([0 1 1 0 0],[0 0 1 1 0]);disp('Mux')
  "pd{2,1}" : Outport
      mask Display: e = 0.06;c1 = [120 230 180]/255;c2 = ([120 230 180]+0)/(256+128);c3 = ([120 230 180]+128)/(256+128);patch([0 1 1 0],[0 0 1 1],c1);patch([0 1 1 1-e 1-e 0+e],[0 0 1 1-e 0+e 0+e],c2);patch([0 0 1 1-e 0+e 0+e],[0 1 1 1-e 1-e 0+e],c3);plot([0 1 1 0 0],[0 0 1 1 0]);
  wires:
  "p{2}"/1 -> mux/1
  mux/1 -> "pd{2,1}"/1
